simulink model "Zadatak1a_PID"  (R2020b)
settings: Solver=VariableStepAuto  StartTime=0.0  StopTime=300.0  RelTol=1e-3
values from neighbouring files (symbols this model uses):
  Kp = (1.2*T0)/(K0*tau)    (= 4.31848525306)    [Zadatak1a_PID_skripta.m]
  T = 0.01    [Zadatak1a_PID_skripta.m]
  Td = 0.5*tau    (= 0.535)    [Zadatak1a_PID_skripta.m]
  Ti = 2*tau    (= 2.14)    [Zadatak1a_PID_skripta.m]
libraries: simulink x1
settings Model: Creator=user  LastModifiedBy=user

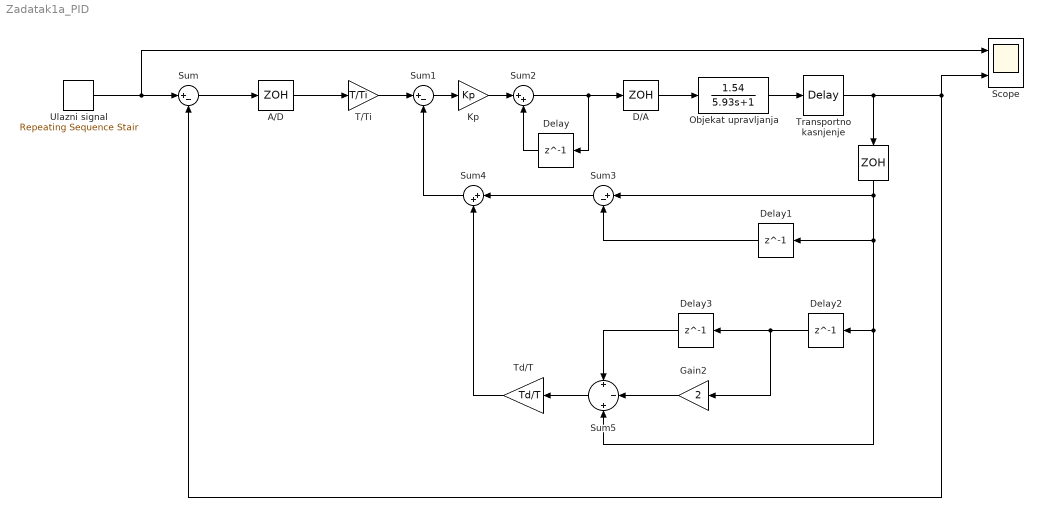
== system Zadatak1a_PID ==
  " " : ZeroOrderHold  SampleTime=0.01
  A/D : ZeroOrderHold  SampleTime=0.01
  D/A : ZeroOrderHold  SampleTime=0.01
  Delay{,1..3} (4 alike) : Delay  DelayLength=1
  Gain2 : Gain  Gain=2
  Kp : Gain  Gain=Kp
  Objekat upravljanja : TransferFcn  Numerator=[1.54]  Denominator=[5.93 1]
  Scope : Scope  NumInputPorts=2
  Sum : Sum  Inputs=|+-
  Sum1 : Sum  Inputs=|+-
  Sum2 : Sum  Inputs=|++
  Sum3 : Sum  Inputs=|+-
  Sum4 : Sum  Inputs=|++
  Sum5 : Sum  Inputs=+|-|+
  T/Ti : Gain  Gain=T/Ti
  Td/T : Gain  Gain=Td/T
  Transportno kasnjenje : TransportDelay  DelayTime=1.07
  Ulazni signal : simulink/Sources/Repeating Sequence Stair  OutValues=[3 1 -5 2 1].'  tsamp=50  OutMin=[]  OutMax=[]  OutDataTypeStr=double  OutputDataTypeScalingMode=double  OutDataType=fixdt(0,8)  ConRadixGroup=Best Precision: Vector-wise  OutScaling=2^-12
  wires:
  Ulazni signal/1 -> Scope/1, Sum/1
  Sum2/1 -> Delay/1, D/A/1
  Sum3/1 -> Sum4/1
  Sum/1 -> A/D/1
  Sum5/1 -> Td/T/1
  Sum1/1 -> Kp/1
  Sum4/1 -> Sum1/2
  " "/1 -> Sum5/3, Delay2/1, Delay1/1, Sum3/1
  Transportno kasnjenje/1 -> Sum/2, Scope/2, " "/1
  T/Ti/1 -> Sum1/1
  Gain2/1 -> Sum5/2
  Delay2/1 -> Delay3/1, Gain2/1
  D/A/1 -> Objekat upravljanja/1
  Delay1/1 -> Sum3/2
  Kp/1 -> Sum2/1
  Delay3/1 -> Sum5/1
  Delay/1 -> Sum2/2
  Td/T/1 -> Sum4/2
  A/D/1 -> T/Ti/1
  Objekat upravljanja/1 -> Transportno kasnjenje/1
